simulink model "FlWtDet_DD"  (R2016b)
settings: configuration reference "CodeGenConfigSet" (kept outside this file)
values from neighbouring files (symbols this model uses):
  FlWLmp_O_D_ATS = Calibration.Parameter    [init_FlWtDet_DD.m]
  FlWLmp_stPsDiaDisbl_C = Calibration.Parameter    [init_FlWtDet_DD.m]
  FlWLmp_stPsDisbl_C = Calibration.Parameter    [init_FlWtDet_DD.m]
  SigTst_swtFlWLmp_C = Calibration.Parameter    [init_FlWtDet_DD.m]
undefined symbols (not defined in the file or in its folder): Switch_conv
settings Model: Creator=Wei Liang  LastModifiedBy=Wei Liang
settings ConfigSetRef: SourceLocation=Base Workspace

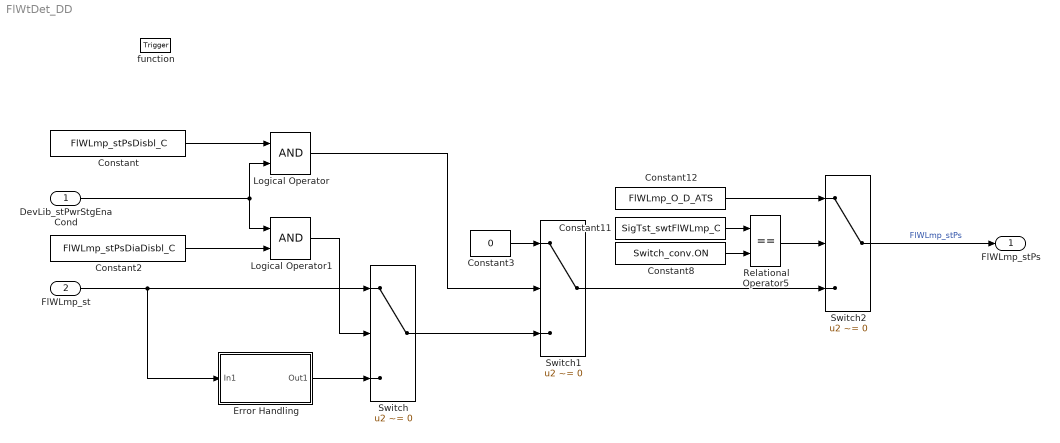
== system FlWtDet_DD ==
  DevLib_stPwrStgEnaCond : Inport  Description=Control unit status relevant to power stage deactivation/error diagnosis  OutMin=0  OutMax=65535  OutDataTypeStr=State_uint16
  FlWLmp_st : Inport  Description=Status of Water Level Indication lamp  Port=2  OutMin=0  OutMax=1  OutDataTypeStr=boolean
  function : TriggerPort  TriggerType=function-call  VariantControl=Variant
  Constant : Constant  Value=FlWLmp_stPsDisbl_C
  Constant11 : Constant  Value=SigTst_swtFlWLmp_C  SampleTime=-1
  Constant12 : Constant  Value=FlWLmp_O_D_ATS  SampleTime=-1
  Constant2 : Constant  Value=FlWLmp_stPsDiaDisbl_C
  Constant3 : Constant  Value=0  OutDataTypeStr=Inherit: Inherit via back propagation
  Constant8 : Constant  Value=Switch_conv.ON  OutDataTypeStr=Inherit: Inherit via back propagation
  Error Handling : Subsystem
  Logical Operator : Logic  AllPortsSameDT=off  OutDataTypeStr=boolean
  Logical Operator1 : Logic  AllPortsSameDT=off  OutDataTypeStr=boolean
  Relational Operator5 : RelationalOperator  Operator===  OutDataTypeStr=boolean  RndMeth=Simplest  InputSameDT=on
  Switch : Switch  Criteria=u2 ~= 0
  Switch1 : Switch  Criteria=u2 ~= 0
  Switch2 : Switch  Criteria=u2 ~= 0
  FlWLmp_stPs : Outport  Description=Status of the power stage for the indication lamp  OutMin=0  OutMax=1  OutDataTypeStr=boolean
  wires:
  Constant/1 -> Logical Operator/1
  DevLib_stPwrStgEnaCond/1 -> Logical Operator1/1, Logical Operator/2
  Constant2/1 -> Logical Operator1/2
  FlWLmp_st/1 -> Error Handling/1(In1), Switch/1
  Error Handling/1(Out1) -> Switch/3
  Logical Operator1/1 -> Switch/2
  Logical Operator/1 -> Switch1/2
  Constant3/1 -> Switch1/1
  Switch/1 -> Switch1/3
  Switch1/1 -> Switch2/3
  Switch2/1 -> FlWLmp_stPs/1  "FlWLmp_stPs"
  Constant12/1 -> Switch2/1
  Constant11/1 -> Relational Operator5/1
  Constant8/1 -> Relational Operator5/2
  Relational Operator5/1 -> Switch2/2

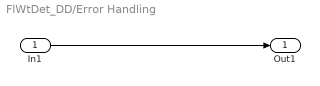
== system FlWtDet_DD/Error Handling ==
  In1 : Inport
  Out1 : Outport
  wires:
  In1/1 -> Out1/1
